simulink model "foswec2Mooring"  (R2025a)
settings: Solver=ode4  StartTime=0  StopTime=100  FixedStep=0.005  MaxStep=0.005  RelTol=1e-3  EnableMultiTasking=on
undefined symbols (not defined in the file or in its folder): body, constraint, mooring, pto
libraries: WECSim_Lib_Body_Elements x3, WECSim_Lib_Moorings x2, WECSim_Lib_PTOs x2, WECSim_Lib_Constraints x1, WECSim_Lib_Frames x1
settings Model: Creator=mlawson  LastModifiedBy=jtgrasb
settings SolverCC: ZeroCrossControl=DisableAll  AlgebraicLoopSolver=LineSearch  AutoInsertRateTranBlk=on
settings DataIOCC: SaveFormat=Array  SaveOutput=off  SaveTime=off  ReturnWorkspaceOutputs=off
settings OptimizationCC: LifeSpan=inf  SimCompilerOptimization=on
settings DebuggingCC: MergeDetectMultiDrivingBlocksExec=none  SolverPrmCheckMsg=warning  UnconnectedInputMsg=warning  UnconnectedOutputMsg=warning  UnconnectedLineMsg=warning  AllowSymbolicDim=off  StateNameClashWarn=warning  SFUnexpectedBacktrackingDiag=warning  SFNoUnconditionalDefaultTransitionDiag=warning  SFExecutionAtInitializationDiag=none  ArithmeticOperatorsInVariantConditions=warning
settings HardwareCC: ProdBitPerPointer=32.0  ProdBitPerSizeT=32.0  ProdBitPerPtrDiffT=32.0  ProdLargestAtomicFloat=None  ProdIntDivRoundTo=Undefined  ProdEndianess=Unspecified  ProdWordSize=32.0  ProdHWDeviceType=32-bit Generic
settings ModelReferenceCC: EnableRefExpFcnMdlSchedulingChecks=on  PropagateSignalLabelsOutOfModel=off
settings SFSimCC: SimUseLocalCustomCode=off  CustomCodeUndefinedFunction=UseInterfaceOnly
settings RTWCC: RTWUseLocalCustomCode=off  GPUComputeCapability=3.5  DLArmComputeVersion=19.05
settings CodeAppCC: StateflowObjectComments=on
settings GRTTargetCC: TargetLangStandard=C89/C90 (ANSI)
settings ConfigComp: CovMetricSettings=dw  CovSaveCumulativeToWorkspaceVar=on  CovSaveSingleToWorkspaceVar=on  CovExternalEMLEnable=off  CovSFcnEnable=off
settings SimscapeCC: SimscapeNormalizeSystem=off
settings ConfigurationSet: Description=SimMechanics 2G
settings ExplorerConfigSet: InternalSimMechanicsExplorerSettings="<ExplorerConfiguration><canonicalview>default</canonicalview><TilePanel><TileInfo><Tiles Columns=\"1\" Count=\"1\" Rows=\"1\"><Column Left=\"2\" Weight=\"1\"/><Column Left=\"1335\"/><Row Top=\"2\" Weight=\"1\"/><Row Top=\"911\"/><Tile Height=\"1\" Width=\"1\" X=\"0\" Y=\"0\"/></Tiles></TileInfo><SceneInfo><SceneViewer><BGColor><R>0.60000002384185791</R><G>0.60000002384185791</G><B>0.60000002384185791</B></BGColor><Camera><Position><X>365.37645888990272</X><Y>-369.82486814446582</Y><Z>359.64809521743916</Z></Position><Center><X>-6.7351450971904585</X><Y>2.2867358426280204</Y><Z>-12.463508769654169</Z></Center><Up><X>-0.40824829046386307</X><Y>0.40824829046386307</Y><Z>0.81649658092772615</Z></Up><Left>-57.820127362122818</Left><Right>57.820127362122818</Right><Bottom>-38.308817187253304</Bottom><Top>38.308817187253304</Top></Camera></SceneViewer></SceneInfo></TilePanel></ExplorerConfiguration>"

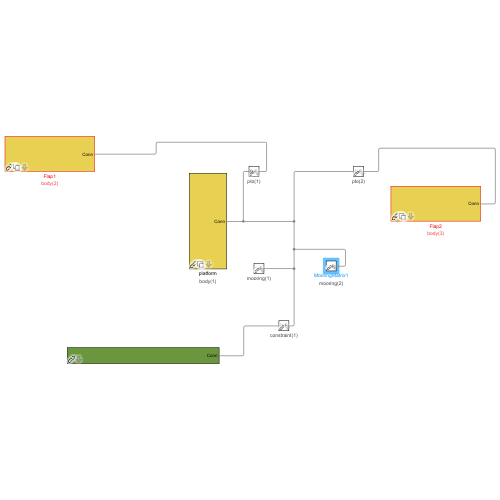
[thumbnail: Simulink's stored preview of the top-level diagram]
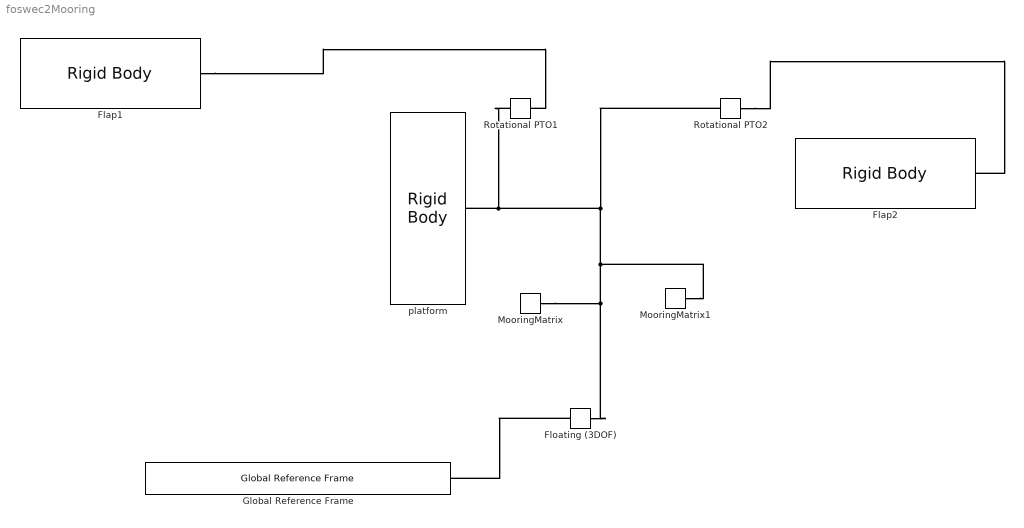
== system foswec2Mooring ==
  Flap1 : WECSim_Lib_Body_Elements/Rigid Body  body=body(2)
  Flap2 : WECSim_Lib_Body_Elements/Rigid Body  body=body(3)
  Floating (3DOF) : WECSim_Lib_Constraints/Floating (3DOF)  constraint=constraint(1)
      settings: AttributesFormatString=%<constraint>
  Global Reference Frame : WECSim_Lib_Frames/Global Reference Frame  waves=waves  simu=simu
  MooringMatrix : WECSim_Lib_Moorings/MooringMatrix  mooring=mooring(1)  loc=0 0 0  preTension=[0 0 0 0 0 0]  stiffness={ '0', '0', '0', '0', '0', '0'; '0', '0', '0', '0', '0', '0'; '0', '0', '0', '0', '0', '0'; '0', '0', '0', '0', '0', '0'; '0', '0', '0', '0', '0', '0'; '0', '0', '0', '0', '0', '0' }  damping={ '0', '0', '0', '0', '0', '0'; '0', '0', '0', '0', '0', '0'; '0', '0', '0', '0', '0', '0'; '0', '0', '0', '0', '0', '0'; '0', '0', '0', '0', '0', '0'; '0', '0', '0', '0', '0', '0' }
      settings: AttributesFormatString=%<mooring>
  MooringMatrix1 : WECSim_Lib_Moorings/MooringMatrix  mooring=mooring(2)  loc=0 0 0  preTension=[0 0 0 0 0 0]  stiffness={ '0', '0', '0', '0', '0', '0'; '0', '0', '0', '0', '0', '0'; '0', '0', '0', '0', '0', '0'; '0', '0', '0', '0', '0', '0'; '0', '0', '0', '0', '0', '0'; '0', '0', '0', '0', '0', '0' }  damping={ '0', '0', '0', '0', '0', '0'; '0', '0', '0', '0', '0', '0'; '0', '0', '0', '0', '0', '0'; '0', '0', '0', '0', '0', '0'; '0', '0', '0', '0', '0', '0'; '0', '0', '0', '0', '0', '0' }
      settings: AttributesFormatString=%<mooring>
  Rotational PTO1 : WECSim_Lib_PTOs/Rotational PTO  pto=pto(1)
      settings: AttributesFormatString=%<pto>
  Rotational PTO2 : WECSim_Lib_PTOs/Rotational PTO  pto=pto(2)
      settings: AttributesFormatString=%<pto>
  platform : WECSim_Lib_Body_Elements/Rigid Body  body=body(1)
  connections:
  Floating (3DOF)/LConn1 -- Global Reference Frame/RConn1
  Floating (3DOF)/RConn1 -- MooringMatrix/LConn1 -- Rotational PTO2/LConn1 -- Rotational PTO1/LConn1 -- platform/RConn1 -- MooringMatrix1/LConn1
  Flap1/RConn1 -- Rotational PTO1/RConn1
  Rotational PTO2/RConn1 -- Flap2/RConn1
